simulink model "AM_DSB_TC_Reciever_that_works"  (R2021b)
settings: Solver=VariableStepAuto  StartTime=0.0  StopTime=inf  RelTol=1e-3
undefined symbols (not defined in the file): fdesignblkfcn, gcbh
libraries: dspsnks4 x1, dspmlti4 x1, sdrrlib x1
settings Model: SimulationMode=accelerator  Creator=Dlope  LastModifiedBy=Dlope

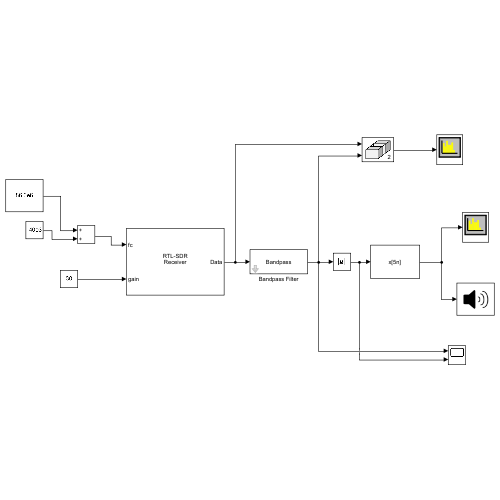
[thumbnail: Simulink's stored preview of the top-level diagram]
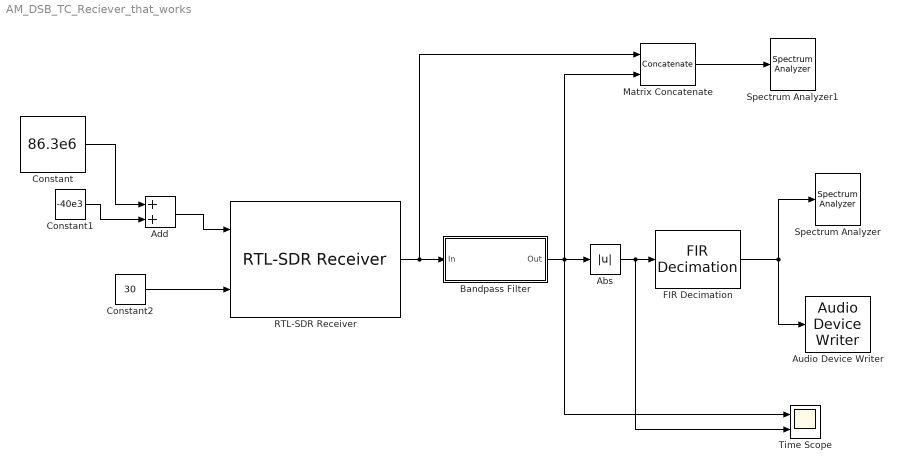
== system AM_DSB_TC_Reciever_that_works ==
  Abs : Abs
  Add : Sum
  Audio Device Writer : dspsnks4/Audio Device Writer  Driver=DirectSound  Device=Speakers (Realtek High Definition Audio(SST))  InheritSampleRate=on  SampleRate=44100  BitDepth=16-bit integer  BufferSize=4096  NumBuffers=10  DefaultOutputChannelMapping=on  OutputChannelMapping=1:2  OutputNumUnderrunSamples=off  DriverIdx=1  DeviceWarnFlag=''
  Bandpass Filter : Subsystem  DialogController=fdesignblkfcn  InitFcn=fdesignblkfcn(gcbh, {'InitFcn'});  mask(Bandpass Filter){}
      mask help: Design a bandpass filter
      settings: CopyFcn=fdesignblkfcn(gcbh, {'CopyFcn'});
      mask Help: helpview(mapfilelocation('dsp'), 'dspbandpassfilter');
      mask Display: disp('Bandpass');
  Constant : Constant  Value=86.3e6
  Constant1 : Constant  Value=-40e3
  Constant2 : Constant  Value=30
  FIR Decimation : dspmlti4/FIR Decimation  FilterSource=Dialog parameters  h=firpm(100, [0 15e3 20e3 (240e3/2)]/(240e3/2), [1 1 0 0], [1 1], 20)  D=5  filtStruct=Direct form  FilterObject=FDECIM  InputProcessing=Columns as channels (frame based)  framing=Allow multirate processing  inputOffset=0  outputBufInitCond=0  roundingMode=Floor  overflowMode=off  firstCoeffDataTypeStr=Inherit: Same word length as input  firstCoeffMin=[]  firstCoeffMax=[]  firstCoeffLastDataTypeStr=Inherit: Same word length as input  outputDataTypeStr=Inherit: Same as accumulator  outputMin=[]  outputMax=[]  outputLastDataTypeStr=Inherit: Same as accumulator
  Matrix Concatenate : Concatenate  Mode=Multidimensional array  ConcatenateDimension=2
  RTL-SDR Receiver : sdrrlib/RTL-SDR Receiver  IPAddress=0  CenterFrequencySource=Input port  CenterFrequency=102.5e6  GainSource=Input port  Gain=0  ADCRate=240e3  FrequencyCorrection=0  LostSamplesOutputPort=off  LatencyOutputPort=off  OutputDataType=single  FrameLength=4096  EnableBurstMode=off  NumFramesInBurst=20  sobjType=sdrr.internal.SDRRTLReceiverSL  dataUDPPort=-1  ctrlUDPPort=-1  subDeviceList=nosubdev  sdrBlockType=SDRBlockTypeSLT.SDRRxBlock  requester=UNUSED_BY_SFCN  sdrExecutionMode=SDRExecutionModeSLT.ExecModeHW  BypassUserLogic=off  DecimatorSelect=DDC decimator  SourceSelect=RF data  SineAmplitude=16000  EnableInternalClock=off  BypassIQBalance=off  IFBandwidth=40e6  ADCRateSource=Dialog  IntermediateFrequency=0  DecimationFactorSource=Dialog  DecimationFactor=512  RFFrequencyIsTunable=logical(1)  SampleTime=(4096)/(240e3)  IFBandwidthSource=Dialog  SineFrequency=30000  BypassDCBlockingFilter=off  IntermediateFrequencySource=Dialog  IQBalanceCoefficients=64  SkipAllHardwareResetAndInitialization=off  EnableIQCalibrationTable=on  CacheIQCalibrationTable=off  EnableOffsetTuning=off  EnableRTLAGC=off  EnableTestMode=off  EnableTunerAGC=off  FrequencyCorrectionSource=Dialog  NumMLBuffers=128  NumUSBBuffers=16  RTLCrystalFrequency=28800000  TunerCrystalFrequency=28800000
      settings: SourceProductBaseCode=RTLSDR
  Spectrum Analyzer : SpectrumAnalyzer
  Spectrum Analyzer1 : SpectrumAnalyzer
  Time Scope : Scope  NumInputPorts=2
  wires:
  Constant2/1 -> RTL-SDR Receiver/2
  Constant/1 -> Add/1
  Constant1/1 -> Add/2
  Add/1 -> RTL-SDR Receiver/1
  RTL-SDR Receiver/1 -> Matrix Concatenate/1, Bandpass Filter/1(In)
  Bandpass Filter/1(Out) -> Time Scope/1, Matrix Concatenate/2, Abs/1
  Abs/1 -> Time Scope/2, FIR Decimation/1
  FIR Decimation/1 -> Spectrum Analyzer/1, Audio Device Writer/1
  Matrix Concatenate/1 -> Spectrum Analyzer1/1

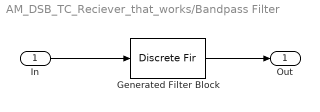
== system AM_DSB_TC_Reciever_that_works/Bandpass Filter ==
  In : Inport
  Generated Filter Block : DiscreteFir  Tag=BlockMethodSubSystem  Coefficients=[0.00243836806543912005 -0.0024904844872335177 0.000829618158798983252 0.000757639909411921475 -0.00297439999954761608 -0.00569567554311764795 -0.00287769587371432354 0.00202335772559120858 0.00233106594051533207 -0.000272122046722700274 0.00129898079076306108 0.00555508782838592344 0.0037368666021221149 -0.0037077560769040222 -0.00613059502047848173 -0.00156733498646652791 -0.000645419817557826283 -0.00588533303396905367 -0.00497548071923390508 0.00605849467576978929 0.012134568108140736 0.00468287519693485164 -0.00196343029761658801 0.00305830740492443829 0.00523359569682744878 -0.00815203734622665065 -0.0196345055166754247 -0.00950525822702418671 0.0068404420787941296 0.00478878751753837248 -0.00332884812683291367 0.00909523350079552428 0.0276394504169403914 0.0161920213367104625 -0.0150761219722256711 -0.0210983733622466876 -0.00274044951834618742 -0.00715859816730031549 -0.0348113060828855597 -0.0258326425539628125 0.0299326964811326528 0.0565084056002555096 0.019341104119483532 -0.00294076064128453085 0.0397881049420063804 0.0472987256841347348 -0.0761641288587477649 -0.207207484433210382 -0.126102083904938628 0.14072053470827206 0.291759208615674559 0.14072053470827206 -0.126102083904938628 -0.207207484433210382 -0.0761641288587477649 0.0472987256841347348 0.0397881049420063804 -0.00294076064128453085 0.019341104119483532 0.0565084056002555096 0.0299326964811326528 -0.0258326425539628125 -0.0348113060828855597 -0.00715859816730031549 -0.00274044951834618742 -0.0210983733622466876 -0.0150761219722256711 0.0161920213367104625 0.0276394504169403914 0.00909523350079552428 -0.00332884812683291367 0.00478878751753837248 0.0068404420787941296 -0.00950525822702418671 -0.0196345055166754247 -0.00815203734622665065 0.00523359569682744878 0.00305830740492443829 -0.00196343029761658801 0.00468287519693485164 0.012134568108140736 0.00605849467576978929 -0.00497548071923390508 -0.00588533303396905367 -0.000645419817557826283 -0.00156733498646652791 -0.00613059502047848173 -0.0037077560769040222 0.0037368666021221149 0.00555508782838592344 0.00129898079076306108 -0.000272122046722700274 0.00233106594051533207 0.00202335772559120858 -0.00287769587371432354 -0.00569567554311764795 -0.00297439999954761608 0.000757639909411921475 0.000829618158798983252 -0.0024904844872335177 0.00243836806543912005]  InputProcessing=Columns as channels (frame based)
  Out : Outport  VectorParamsAs1DForOutWhenUnconnected=off
  wires:
  In/1 -> Generated Filter Block/1
  Generated Filter Block/1 -> Out/1
